simulink model "inverse_velocity_model"  (R2020a)
settings: Solver=VariableStepAuto  StartTime=0.0  StopTime=10.0  RelTol=1e-3
settings Model: Creator=Lord  LastModifiedBy=ElMousel

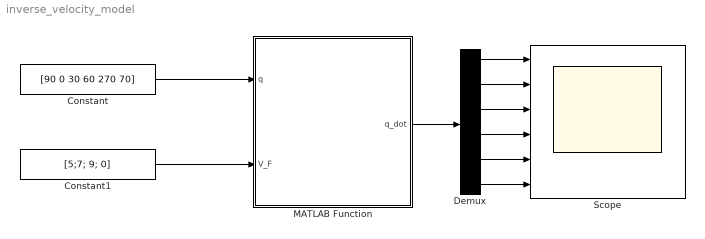
== system inverse_velocity_model ==
  Constant : Constant  Value=[90 0 30 60 270 70]
  Constant1 : Constant  Value=[5;7; 9; 0]
  Demux : Demux  Outputs=6
  MATLAB Function : MATLAB Function  TreatAsAtomicUnit=on
  Scope : Scope  NumInputPorts=6
  wires:
  Constant/1 -> MATLAB Function/1(q)
  Constant1/1 -> MATLAB Function/2(V_F)
  Demux/1 -> Scope/1
  Demux/2 -> Scope/2
  Demux/3 -> Scope/3
  Demux/4 -> Scope/4
  Demux/5 -> Scope/5
  Demux/6 -> Scope/6
  MATLAB Function/1(q_dot) -> Demux/1

== matlab function inverse_velocity_model/MATLAB Function ==
  data: q input; q_dot output; V_F input
function q_dot=inverse_velocity_model(q,V_F)
%j_inv= inverse_jacobian_matrix(q)
 J=jacobian_matrix_num(q);
 r=rank(J)
 b=zeros(4,6);
 q_dot=zeros(6,1);
 for i=1:4
     for j =1:6
         b(i,j)=J(i,j);
     end
 end
 a=b
 r=rank(a)       
%  [RB,p]= rref(J);

j_inv=pinv(b);
x=V_F;
 q_dot=j_inv*V_F

end
